simulink model "QD2_MissionCtrl_Swarm_6x_R2021a"  (R2021a)
settings: Solver=ode2  StartTime=0.0  StopTime=inf  FixedStep=0.001  RelTol=1e-3  EnableMultiTasking=on
undefined symbols (not defined in the file): datetime, Host, localhost, m, qc_get_step_size, saved_data
libraries: quarc_library x64, simulink x19, simulink_extras x1
(part 2 of 3)

== system QD2_MissionCtrl_Swarm_6x_R2021a/MISSION SERVER QDRONE SWARM/Calculate Home Pose V4 ==
  note: This subsystem waits during the first 5 seconds of starting the Mission Server before passing any post measurement.
      | This is to let the initial transient settles down (initialization, communication with the localization system, etc).
      | After the first 5 seconds, this subsystem will latch and pass along the pose measure as the QDrone Home Pose when
      | the ARM signal is received.
      | This home position will reflect whatever pose the user initially places the QDrone in.
      | This is with respect to the Research Studio Frame (RSF).
      |
      | NOTE : The height value of the home pose is the initial measured height PLUS the Home height (m) input value.
  Home height (m) : Inport
  "Pose (m, rad ) [4]" : Inport  Port=2
  Arm(0,1) : Inport  Port=3
  Clock : Clock
  Compare To Constant : simulink/Logic and Bit Operations/Compare To Constant  relop=>  const=5  OutDataTypeStr=boolean
  Constant : Constant  Value=0
  Constant1 : Constant
  Demux : Demux
  Enabled Subsystem : Subsystem  TreatAsAtomicUnit=on
  Logical Operator : Logic  AllPortsSameDT=off  OutDataTypeStr=boolean
  Mux : Mux
  One Shot : quarc_library/Discontinuities/One Shot  trigger_type=Rising edge  redun_pulse=Ignore extraneous pulse  width_source=Specify via dialog  pulse_width=1/qc_get_step_size
      settings: SourceProductName=QUARC Targets
  Selector : Selector  InputPortWidth=6  IndexOptions=Index vector (dialog)  Indices=[1:3,6]  OutputSizes=1
  Sum : Sum
  "Home Pose (m, rad) [4]" : Outport  VectorParamsAs1DForOutWhenUnconnected=off
  wires:
  Constant/1 -> One Shot/2
  Constant1/1 -> One Shot/3
  Arm(0,1)/1 -> One Shot/1
  One Shot/1 -> Logical Operator/2
  "Pose (m, rad ) [4]"/1 -> Selector/1
  Clock/1 -> Compare To Constant/1
  Compare To Constant/1 -> Logical Operator/1
  Logical Operator/1 -> Enabled Subsystem/Enable
  Enabled Subsystem/1("Home Pose (m, rad ) [4]") -> Demux/1
  Demux/1 -> Mux/1
  Demux/2 -> Mux/2
  Demux/4 -> Mux/4
  Demux/3 -> Sum/1
  Sum/1 -> Mux/3
  Home height (m)/1 -> Sum/2
  Mux/1 -> "Home Pose (m, rad) [4]"/1
  Selector/1 -> Enabled Subsystem/1("Pose (m, rad ) [4] ")

== system QD2_MissionCtrl_Swarm_6x_R2021a/MISSION SERVER QDRONE SWARM/Calculate Home Pose V5 ==
  note: This subsystem waits during the first 5 seconds of starting the Mission Server before passing any post measurement.
      | This is to let the initial transient settles down (initialization, communication with the localization system, etc).
      | After the first 5 seconds, this subsystem will latch and pass along the pose measure as the QDrone Home Pose when
      | the ARM signal is received.
      | This home position will reflect whatever pose the user initially places the QDrone in.
      | This is with respect to the Research Studio Frame (RSF).
      |
      | NOTE : The height value of the home pose is the initial measured height PLUS the Home height (m) input value.
  Home height (m) : Inport
  "Pose (m, rad ) [4]" : Inport  Port=2
  Arm(0,1) : Inport  Port=3
  Clock : Clock
  Compare To Constant : simulink/Logic and Bit Operations/Compare To Constant  relop=>  const=5  OutDataTypeStr=boolean
  Constant : Constant  Value=0
  Constant1 : Constant
  Demux : Demux
  Enabled Subsystem : Subsystem  TreatAsAtomicUnit=on
  Logical Operator : Logic  AllPortsSameDT=off  OutDataTypeStr=boolean
  Mux : Mux
  One Shot : quarc_library/Discontinuities/One Shot  trigger_type=Rising edge  redun_pulse=Ignore extraneous pulse  width_source=Specify via dialog  pulse_width=1/qc_get_step_size
      settings: SourceProductName=QUARC Targets
  Selector : Selector  InputPortWidth=6  IndexOptions=Index vector (dialog)  Indices=[1:3,6]  OutputSizes=1
  Sum : Sum
  "Home Pose (m, rad) [4]" : Outport  VectorParamsAs1DForOutWhenUnconnected=off
  wires:
  Constant/1 -> One Shot/2
  Constant1/1 -> One Shot/3
  Arm(0,1)/1 -> One Shot/1
  One Shot/1 -> Logical Operator/2
  "Pose (m, rad ) [4]"/1 -> Selector/1
  Clock/1 -> Compare To Constant/1
  Compare To Constant/1 -> Logical Operator/1
  Logical Operator/1 -> Enabled Subsystem/Enable
  Enabled Subsystem/1("Home Pose (m, rad ) [4]") -> Demux/1
  Demux/1 -> Mux/1
  Demux/2 -> Mux/2
  Demux/4 -> Mux/4
  Demux/3 -> Sum/1
  Sum/1 -> Mux/3
  Home height (m)/1 -> Sum/2
  Mux/1 -> "Home Pose (m, rad) [4]"/1
  Selector/1 -> Enabled Subsystem/1("Pose (m, rad ) [4] ")

== system QD2_MissionCtrl_Swarm_6x_R2021a/MISSION SERVER QDRONE SWARM/Calculate Home Pose V6 ==
  note: This subsystem waits during the first 5 seconds of starting the Mission Server before passing any post measurement.
      | This is to let the initial transient settles down (initialization, communication with the localization system, etc).
      | After the first 5 seconds, this subsystem will latch and pass along the pose measure as the QDrone Home Pose when
      | the ARM signal is received.
      | This home position will reflect whatever pose the user initially places the QDrone in.
      | This is with respect to the Research Studio Frame (RSF).
      |
      | NOTE : The height value of the home pose is the initial measured height PLUS the Home height (m) input value.
  Home height (m) : Inport
  "Pose (m, rad ) [4]" : Inport  Port=2
  Arm(0,1) : Inport  Port=3
  Clock : Clock
  Compare To Constant : simulink/Logic and Bit Operations/Compare To Constant  relop=>  const=5  OutDataTypeStr=boolean
  Constant : Constant  Value=0
  Constant1 : Constant
  Demux : Demux
  Enabled Subsystem : Subsystem  TreatAsAtomicUnit=on
  Logical Operator : Logic  AllPortsSameDT=off  OutDataTypeStr=boolean
  Mux : Mux
  One Shot : quarc_library/Discontinuities/One Shot  trigger_type=Rising edge  redun_pulse=Ignore extraneous pulse  width_source=Specify via dialog  pulse_width=1/qc_get_step_size
      settings: SourceProductName=QUARC Targets
  Selector : Selector  InputPortWidth=6  IndexOptions=Index vector (dialog)  Indices=[1:3,6]  OutputSizes=1
  Sum : Sum
  "Home Pose (m, rad) [4]" : Outport  VectorParamsAs1DForOutWhenUnconnected=off
  wires:
  Constant/1 -> One Shot/2
  Constant1/1 -> One Shot/3
  Arm(0,1)/1 -> One Shot/1
  One Shot/1 -> Logical Operator/2
  "Pose (m, rad ) [4]"/1 -> Selector/1
  Clock/1 -> Compare To Constant/1
  Compare To Constant/1 -> Logical Operator/1
  Logical Operator/1 -> Enabled Subsystem/Enable
  Enabled Subsystem/1("Home Pose (m, rad ) [4]") -> Demux/1
  Demux/1 -> Mux/1
  Demux/2 -> Mux/2
  Demux/4 -> Mux/4
  Demux/3 -> Sum/1
  Sum/1 -> Mux/3
  Home height (m)/1 -> Sum/2
  Mux/1 -> "Home Pose (m, rad) [4]"/1
  Selector/1 -> Enabled Subsystem/1("Pose (m, rad ) [4] ")

== system QD2_MissionCtrl_Swarm_6x_R2021a/MISSION SERVER QDRONE SWARM/Calculate Home Pose V7 ==
  note: This subsystem waits during the first 5 seconds of starting the Mission Server before passing any post measurement.
      | This is to let the initial transient settles down (initialization, communication with the localization system, etc).
      | After the first 5 seconds, this subsystem will latch and pass along the pose measure as the QDrone Home Pose when
      | the ARM signal is received.
      | This home position will reflect whatever pose the user initially places the QDrone in.
      | This is with respect to the Research Studio Frame (RSF).
      |
      | NOTE : The height value of the home pose is the initial measured height PLUS the Home height (m) input value.
  Home height (m) : Inport
  "Pose (m, rad ) [4]" : Inport  Port=2
  Arm(0,1) : Inport  Port=3
  Clock : Clock
  Compare To Constant : simulink/Logic and Bit Operations/Compare To Constant  relop=>  const=5  OutDataTypeStr=boolean
  Constant : Constant  Value=0
  Constant1 : Constant
  Demux : Demux
  Enabled Subsystem : Subsystem  TreatAsAtomicUnit=on
  Logical Operator : Logic  AllPortsSameDT=off  OutDataTypeStr=boolean
  Mux : Mux
  One Shot : quarc_library/Discontinuities/One Shot  trigger_type=Rising edge  redun_pulse=Ignore extraneous pulse  width_source=Specify via dialog  pulse_width=1/qc_get_step_size
      settings: SourceProductName=QUARC Targets
  Sum : Sum
  "Home Pose (m, rad) [4]" : Outport  VectorParamsAs1DForOutWhenUnconnected=off
  wires:
  Constant/1 -> One Shot/2
  Constant1/1 -> One Shot/3
  Arm(0,1)/1 -> One Shot/1
  One Shot/1 -> Logical Operator/2
  "Pose (m, rad ) [4]"/1 -> Enabled Subsystem/1("Pose (m, rad ) [4] ")
  Clock/1 -> Compare To Constant/1
  Compare To Constant/1 -> Logical Operator/1
  Logical Operator/1 -> Enabled Subsystem/Enable
  Enabled Subsystem/1("Home Pose (m, rad ) [4]") -> Demux/1
  Demux/1 -> Mux/1
  Demux/2 -> Mux/2
  Demux/4 -> Mux/4
  Demux/3 -> Sum/1
  Sum/1 -> Mux/3
  Home height (m)/1 -> Sum/2
  Mux/1 -> "Home Pose (m, rad) [4]"/1

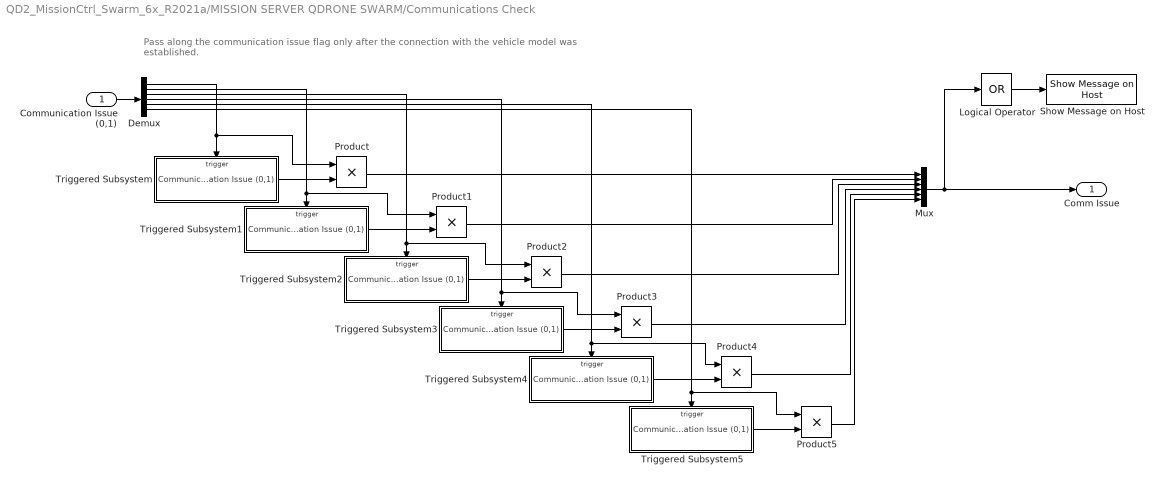
== system QD2_MissionCtrl_Swarm_6x_R2021a/MISSION SERVER QDRONE SWARM/Communications Check ==
  note: Pass along the communication issue flag only after the connection with the vehicle model was established.
  Communication Issue (0,1) : Inport
  Demux : Demux  Outputs=6
  Logical Operator : Logic  Operator=OR  Inputs=1  AllPortsSameDT=off  OutDataTypeStr=boolean
  Mux : Mux  Inputs=6
  Product{,1..5} (6 alike) : Product
  Show Message on Host : quarc_library/Sinks/Error Handling/Show Message on Host  message_type=Fixed error message  message_icon=Warning  message=Mission Server: Communication Issue with a QDrone
      settings: AttributesFormatString="\"%<message>\""  SourceProductName=QUARC Targets
  Triggered Subsystem : Subsystem  TreatAsAtomicUnit=on
  Triggered Subsystem1 : Subsystem  TreatAsAtomicUnit=on
  Triggered Subsystem2 : Subsystem  TreatAsAtomicUnit=on
  Triggered Subsystem3 : Subsystem  TreatAsAtomicUnit=on
  Triggered Subsystem4 : Subsystem  TreatAsAtomicUnit=on
  Triggered Subsystem5 : Subsystem  TreatAsAtomicUnit=on
  Comm Issue : Outport  VectorParamsAs1DForOutWhenUnconnected=off
  wires:
  Communication Issue (0,1)/1 -> Demux/1
  Demux/1 -> Product/1, Triggered Subsystem/Trigger
  Demux/2 -> Product1/1, Triggered Subsystem1/Trigger
  Demux/3 -> Product2/1, Triggered Subsystem2/Trigger
  Demux/4 -> Product3/1, Triggered Subsystem3/Trigger
  Demux/5 -> Product4/1, Triggered Subsystem4/Trigger
  Demux/6 -> Product5/1, Triggered Subsystem5/Trigger
  Triggered Subsystem/1(Communication Issue (0,1)) -> Product/2
  Triggered Subsystem5/1(Communication Issue (0,1)) -> Product5/2
  Triggered Subsystem4/1(Communication Issue (0,1)) -> Product4/2
  Triggered Subsystem3/1(Communication Issue (0,1)) -> Product3/2
  Triggered Subsystem2/1(Communication Issue (0,1)) -> Product2/2
  Triggered Subsystem1/1(Communication Issue (0,1)) -> Product1/2
  Product4/1 -> Mux/5
  Product3/1 -> Mux/4
  Product5/1 -> Mux/6
  Product2/1 -> Mux/3
  Product1/1 -> Mux/2
  Product/1 -> Mux/1
  Mux/1 -> Logical Operator/1, Comm Issue/1
  Logical Operator/1 -> Show Message on Host/1

== system QD2_MissionCtrl_Swarm_6x_R2021a/MISSION SERVER QDRONE SWARM/Extract Vehicle Data 1 ==
  Optitrack Data : Inport
  Vehicle ID : Inport  Port=2
  Data Type Conversion10 : DataTypeConversion
  Data Type Conversion11 : DataTypeConversion
  Data Type Conversion9 : DataTypeConversion
  Extract Object Data : MATLAB Function  TreatAsAtomicUnit=on
  Mux1 : Mux  Inputs=3
  Reshape : Reshape
  Reshape1 : Reshape
  Reshape2 : Reshape
  Vehicle Data : Outport  VectorParamsAs1DForOutWhenUnconnected=off
  wires:
  Reshape2/1 -> Data Type Conversion9/1
  Reshape1/1 -> Data Type Conversion10/1
  Reshape/1 -> Data Type Conversion11/1
  Data Type Conversion9/1 -> Mux1/3
  Data Type Conversion10/1 -> Mux1/2
  Data Type Conversion11/1 -> Mux1/1
  Extract Object Data/2(orientation) -> Reshape1/1
  Extract Object Data/3(tracking) -> Reshape2/1
  Extract Object Data/1(position) -> Reshape/1
  Mux1/1 -> Vehicle Data/1
  Optitrack Data/1 -> Extract Object Data/1(data)
  Vehicle ID/1 -> Extract Object Data/2(index)

== system QD2_MissionCtrl_Swarm_6x_R2021a/MISSION SERVER QDRONE SWARM/Extract Vehicle Data 2 ==
  Optitrack Data : Inport
  Vehicle ID : Inport  Port=2
  Data Type Conversion10 : DataTypeConversion
  Data Type Conversion11 : DataTypeConversion
  Data Type Conversion9 : DataTypeConversion
  Extract Object Data : MATLAB Function  TreatAsAtomicUnit=on
  Mux1 : Mux  Inputs=3
  Reshape : Reshape
  Reshape1 : Reshape
  Reshape2 : Reshape
  Vehicle Data : Outport  VectorParamsAs1DForOutWhenUnconnected=off
  wires:
  Vehicle ID/1 -> Extract Object Data/2(index)
  Optitrack Data/1 -> Extract Object Data/1(data)
  Mux1/1 -> Vehicle Data/1
  Extract Object Data/1(position) -> Reshape/1
  Extract Object Data/3(tracking) -> Reshape2/1
  Extract Object Data/2(orientation) -> Reshape1/1
  Data Type Conversion11/1 -> Mux1/1
  Data Type Conversion10/1 -> Mux1/2
  Data Type Conversion9/1 -> Mux1/3
  Reshape/1 -> Data Type Conversion11/1
  Reshape1/1 -> Data Type Conversion10/1
  Reshape2/1 -> Data Type Conversion9/1

== system QD2_MissionCtrl_Swarm_6x_R2021a/MISSION SERVER QDRONE SWARM/Extract Vehicle Data 3 ==
  Optitrack Data : Inport
  Vehicle ID : Inport  Port=2
  Data Type Conversion10 : DataTypeConversion
  Data Type Conversion11 : DataTypeConversion
  Data Type Conversion9 : DataTypeConversion
  Extract Object Data : MATLAB Function  TreatAsAtomicUnit=on
  Mux1 : Mux  Inputs=3
  Reshape : Reshape
  Reshape1 : Reshape
  Reshape2 : Reshape
  Vehicle Data : Outport  VectorParamsAs1DForOutWhenUnconnected=off
  wires:
  Vehicle ID/1 -> Extract Object Data/2(index)
  Optitrack Data/1 -> Extract Object Data/1(data)
  Mux1/1 -> Vehicle Data/1
  Extract Object Data/1(position) -> Reshape/1
  Extract Object Data/3(tracking) -> Reshape2/1
  Extract Object Data/2(orientation) -> Reshape1/1
  Data Type Conversion11/1 -> Mux1/1
  Data Type Conversion10/1 -> Mux1/2
  Data Type Conversion9/1 -> Mux1/3
  Reshape/1 -> Data Type Conversion11/1
  Reshape1/1 -> Data Type Conversion10/1
  Reshape2/1 -> Data Type Conversion9/1

== system QD2_MissionCtrl_Swarm_6x_R2021a/MISSION SERVER QDRONE SWARM/Extract Vehicle Data 4 ==
  Optitrack Data : Inport
  Vehicle ID : Inport  Port=2
  Data Type Conversion10 : DataTypeConversion
  Data Type Conversion11 : DataTypeConversion
  Data Type Conversion9 : DataTypeConversion
  Extract Object Data : MATLAB Function  TreatAsAtomicUnit=on
  Mux1 : Mux  Inputs=3
  Reshape : Reshape
  Reshape1 : Reshape
  Reshape2 : Reshape
  Vehicle Data : Outport  VectorParamsAs1DForOutWhenUnconnected=off
  wires:
  Reshape2/1 -> Data Type Conversion9/1
  Reshape1/1 -> Data Type Conversion10/1
  Reshape/1 -> Data Type Conversion11/1
  Data Type Conversion9/1 -> Mux1/3
  Data Type Conversion10/1 -> Mux1/2
  Data Type Conversion11/1 -> Mux1/1
  Extract Object Data/2(orientation) -> Reshape1/1
  Extract Object Data/3(tracking) -> Reshape2/1
  Extract Object Data/1(position) -> Reshape/1
  Mux1/1 -> Vehicle Data/1
  Optitrack Data/1 -> Extract Object Data/1(data)
  Vehicle ID/1 -> Extract Object Data/2(index)

== system QD2_MissionCtrl_Swarm_6x_R2021a/MISSION SERVER QDRONE SWARM/Extract Vehicle Data 5 ==
  Optitrack Data : Inport
  Vehicle ID : Inport  Port=2
  Data Type Conversion10 : DataTypeConversion
  Data Type Conversion11 : DataTypeConversion
  Data Type Conversion9 : DataTypeConversion
  Extract Object Data : MATLAB Function  TreatAsAtomicUnit=on
  Mux1 : Mux  Inputs=3
  Reshape : Reshape
  Reshape1 : Reshape
  Reshape2 : Reshape
  Vehicle Data : Outport  VectorParamsAs1DForOutWhenUnconnected=off
  wires:
  Vehicle ID/1 -> Extract Object Data/2(index)
  Optitrack Data/1 -> Extract Object Data/1(data)
  Mux1/1 -> Vehicle Data/1
  Extract Object Data/1(position) -> Reshape/1
  Extract Object Data/3(tracking) -> Reshape2/1
  Extract Object Data/2(orientation) -> Reshape1/1
  Data Type Conversion11/1 -> Mux1/1
  Data Type Conversion10/1 -> Mux1/2
  Data Type Conversion9/1 -> Mux1/3
  Reshape/1 -> Data Type Conversion11/1
  Reshape1/1 -> Data Type Conversion10/1
  Reshape2/1 -> Data Type Conversion9/1

== system QD2_MissionCtrl_Swarm_6x_R2021a/MISSION SERVER QDRONE SWARM/Extract Vehicle Data 6 ==
  Optitrack Data : Inport
  Vehicle ID : Inport  Port=2
  Data Type Conversion10 : DataTypeConversion
  Data Type Conversion11 : DataTypeConversion
  Data Type Conversion9 : DataTypeConversion
  Extract Object Data : MATLAB Function  TreatAsAtomicUnit=on
  Mux1 : Mux  Inputs=3
  Reshape : Reshape
  Reshape1 : Reshape
  Reshape2 : Reshape
  Vehicle Data : Outport  VectorParamsAs1DForOutWhenUnconnected=off
  wires:
  Reshape2/1 -> Data Type Conversion9/1
  Reshape1/1 -> Data Type Conversion10/1
  Reshape/1 -> Data Type Conversion11/1
  Data Type Conversion9/1 -> Mux1/3
  Data Type Conversion10/1 -> Mux1/2
  Data Type Conversion11/1 -> Mux1/1
  Extract Object Data/2(orientation) -> Reshape1/1
  Extract Object Data/3(tracking) -> Reshape2/1
  Extract Object Data/1(position) -> Reshape/1
  Mux1/1 -> Vehicle Data/1
  Optitrack Data/1 -> Extract Object Data/1(data)
  Vehicle ID/1 -> Extract Object Data/2(index)

== system QD2_MissionCtrl_Swarm_6x_R2021a/MISSION SERVER QDRONE SWARM/Extract Vehicle Data 7 ==
  Optitrack Data : Inport
  Vehicle ID : Inport  Port=2
  Data Type Conversion10 : DataTypeConversion
  Data Type Conversion11 : DataTypeConversion
  Data Type Conversion9 : DataTypeConversion
  Extract Object Data : MATLAB Function  TreatAsAtomicUnit=on
  Mux1 : Mux  Inputs=3
  Reshape : Reshape
  Reshape1 : Reshape
  Reshape2 : Reshape
  Vehicle Data : Outport  VectorParamsAs1DForOutWhenUnconnected=off
  wires:
  Reshape2/1 -> Data Type Conversion9/1
  Reshape1/1 -> Data Type Conversion10/1
  Reshape/1 -> Data Type Conversion11/1
  Data Type Conversion9/1 -> Mux1/3
  Data Type Conversion10/1 -> Mux1/2
  Data Type Conversion11/1 -> Mux1/1
  Extract Object Data/2(orientation) -> Reshape1/1
  Extract Object Data/3(tracking) -> Reshape2/1
  Extract Object Data/1(position) -> Reshape/1
  Mux1/1 -> Vehicle Data/1
  Optitrack Data/1 -> Extract Object Data/1(data)
  Vehicle ID/1 -> Extract Object Data/2(index)

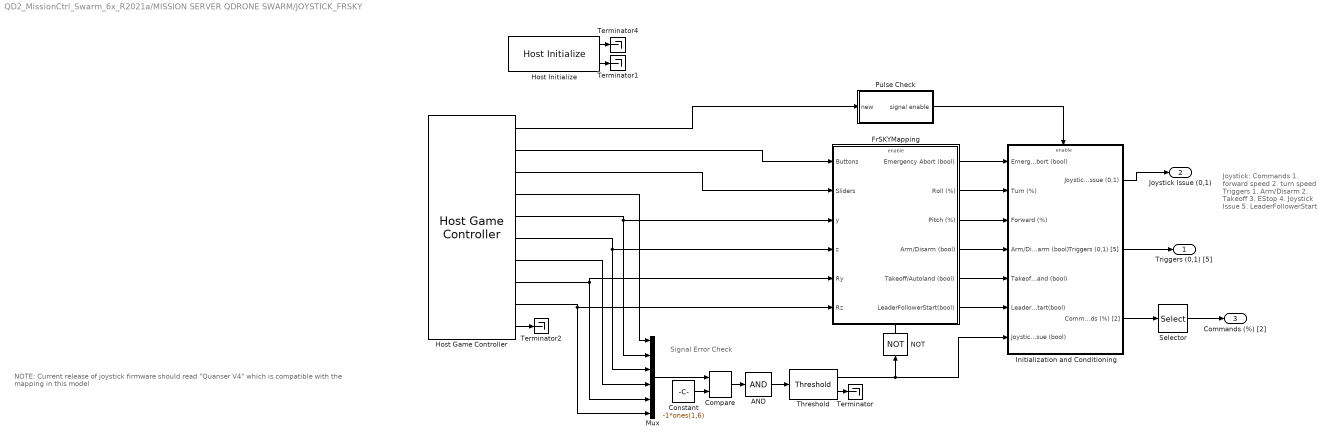
== system QD2_MissionCtrl_Swarm_6x_R2021a/MISSION SERVER QDRONE SWARM/JOYSTICK_FRSKY ==
  note: Signal Error Check
  note: NOTE: Current release of joystick firmware should read "Quanser V4" which is compatible with the mapping in this model
  note: Joystick:
      | Commands
      | 	1. forward speed
      | 	2. turn speed
      | Triggers
      | 	1. Arm/Disarm
      | 	2. Takeoff
      | 	3. EStop
      | 	4. Joystick Issue
      |
      | 	5. LeaderFollowerStart
  AND : Logic  Inputs=1  AllPortsSameDT=off  OutDataTypeStr=boolean
  Compare : quarc_library/Logic Operations/Compare  operator===  output_data_type=boolean
      settings: SourceProductName=QUARC Targets
  Constant : Constant  Value=-1*ones(1,6)
  FrSKYMapping : Subsystem
  Host Game Controller : quarc_library/Devices/Peripherals/Host/Host Game Controller  object_name=Host-1  controller=1  buffer_size=20  deadzone=[]  saturation=[]  sample_time=qc_get_step_size  auto_center=off  enabled=on  debug_mode=off
      settings: SourceProductName=QUARC Targets
  Host Initialize : quarc_library/Devices/Peripherals/Host/Host Initialize  object_name=Host-1  uri_source=Specify via dialog (do not evaluate)  uri=tcpip://localhost:18005  send_buffer_size=1000  receive_buffer_size=1000  thread_priority=0  run_client=on  use_window=off  window_position=[]  sample_time=qc_get_step_size  active=on
      settings: AttributesFormatString="\"tcpip://localhost:18005\""  SourceProductName=QUARC Targets
  Initialization and Conditioning : Subsystem  TreatAsAtomicUnit=on
  Mux : Mux  Inputs=6
  NOT : Logic  Operator=NOT  IconShape=distinctive  AllPortsSameDT=off  OutDataTypeStr=boolean
  Pulse Check : Subsystem  TreatAsAtomicUnit=on
  Selector : Selector  InputPortWidth=2  IndexOptions=Index vector (dialog)  Indices=[2 1]  OutputSizes=1
  Terminator{,1..2,4} (4 alike) : Terminator
  Threshold : quarc_library/Discontinuities/Threshold  operator=>=  param_src=Specify via dialog  threshold=0.5  duration=0.2
      settings: SourceProductName=QUARC Targets
  Triggers (0,1) [5] : Outport  VectorParamsAs1DForOutWhenUnconnected=off
  Joystick Issue (0,1) : Outport  Port=2  VectorParamsAs1DForOutWhenUnconnected=off
  Commands (%) [2] : Outport  Port=3  VectorParamsAs1DForOutWhenUnconnected=off
  wires:
  Host Game Controller/10 -> Terminator2/1
  Pulse Check/1(signal enable) -> Initialization and Conditioning/Enable
  Host Initialize/1 -> Terminator4/1
  FrSKYMapping/4("Arm/Disarm (bool) ") -> Initialization and Conditioning/4(Arm/Disarm (bool))
  Host Initialize/2 -> Terminator1/1
  FrSKYMapping/5(Takeoff/Autoland (bool)) -> Initialization and Conditioning/5(Takeoff/AutoLand (bool))
  Host Game Controller/7 -> Mux/4
  Host Game Controller/8 -> Mux/5, FrSKYMapping/5(Ry)
  Initialization and Conditioning/3(Commands (%) [2]) -> Selector/1
  Host Game Controller/5 -> Mux/2, FrSKYMapping/3(y)
  Host Game Controller/9 -> Mux/6, FrSKYMapping/6(Rz)
  Host Game Controller/1 -> Pulse Check/1(new)
  Mux/1 -> Compare/1
  Threshold/1 -> NOT/1, Initialization and Conditioning/7(Joystick Issue (bool))
  AND/1 -> Threshold/1
  Host Game Controller/3 -> FrSKYMapping/2(Sliders)
  Threshold/2 -> Terminator/1
  NOT/1 -> FrSKYMapping/Enable
  Constant/1 -> Compare/2
  Host Game Controller/6 -> Mux/3, FrSKYMapping/4(z)
  FrSKYMapping/2(Roll (%)) -> Initialization and Conditioning/2(Turn (%))
  FrSKYMapping/3(Pitch (%)) -> Initialization and Conditioning/3(Forward (%))
  Compare/1 -> AND/1
  FrSKYMapping/1(Emergency Abort (bool)) -> Initialization and Conditioning/1(Emergency Abort (bool))
  Initialization and Conditioning/1(Joystick Issue (0,1)) -> Joystick Issue (0,1)/1
  Initialization and Conditioning/2(Triggers (0,1) [5]) -> Triggers (0,1) [5]/1
  Host Game Controller/4 -> Mux/1
  Host Game Controller/2 -> FrSKYMapping/1(Buttons)
  FrSKYMapping/6(LeaderFollowerStart(bool)) -> Initialization and Conditioning/6(LeaderFollowerStart(bool))
  Selector/1 -> Commands (%) [2]/1

== system QD2_MissionCtrl_Swarm_6x_R2021a/MISSION SERVER QDRONE SWARM/JOYSTICK_SPEKTRUM ==
  note: Throttle
      | Roll
      | Pitch
      | Yaw
  Host Game Controller : quarc_library/Devices/Peripherals/Host/Host Game Controller  object_name=Host-2  controller=1  buffer_size=20  deadzone=[]  saturation=[]  sample_time=qc_get_step_size  auto_center=off  enabled=on  debug_mode=off
      settings: SourceProductName=QUARC Targets
  Host Initialize : quarc_library/Devices/Peripherals/Host/Host Initialize  object_name=Host-2  uri_source=Use external mode communications  uri=tcpip://localhost:18001  send_buffer_size=1000  receive_buffer_size=1000  thread_priority=0  run_client=on  use_window=off  window_position=[]  sample_time=qc_get_step_size  active=on
      settings: SourceProductName=QUARC Targets
  Initialization and Conditioning : Subsystem  TreatAsAtomicUnit=on
  Pulse Check : Subsystem  TreatAsAtomicUnit=on
  Spectrum DXe Mapping : Subsystem
  Terminator{1..4} (4 alike) : Terminator
  Triggers (0,1) [4] : Outport  VectorParamsAs1DForOutWhenUnconnected=off
  Joystick Issue (0,1) : Outport  Port=2  VectorParamsAs1DForOutWhenUnconnected=off
  Commands (%) [4] : Outport  Port=3  VectorParamsAs1DForOutWhenUnconnected=off
  wires:
  Pulse Check/1(signal enable) -> Initialization and Conditioning/Enable
  Host Game Controller/1 -> Pulse Check/1(new), Spectrum DXe Mapping/1(new)
  Initialization and Conditioning/3(Commands (%) [4]) -> Commands (%) [4]/1
  Spectrum DXe Mapping/8(Takeoff/Autoland (bool)) -> Initialization and Conditioning/8(Takeoff/AutoLand (bool))
  Initialization and Conditioning/2(Triggers (0,1) [4]) -> Triggers (0,1) [4]/1
  Spectrum DXe Mapping/2(Emergency Abort (bool)) -> Initialization and Conditioning/2(Emergency Abort (bool))
  Host Game Controller/2 -> Spectrum DXe Mapping/2(buttons)
  Spectrum DXe Mapping/6(Pitch (%)) -> Initialization and Conditioning/6(Pitch (%))
  Spectrum DXe Mapping/4(Throttle (%)) -> Initialization and Conditioning/4(Throttle (%))
  Spectrum DXe Mapping/5(Roll (%)) -> Initialization and Conditioning/5(Roll (%))
  Spectrum DXe Mapping/7("Arm/Disarm (bool) ") -> Initialization and Conditioning/7(Arm/Disarm (bool))
  Spectrum DXe Mapping/3(Yaw (%)) -> Initialization and Conditioning/3(Yaw (%))
  Host Initialize/2 -> Terminator1/1
  Host Initialize/1 -> Terminator4/1
  Host Game Controller/6 -> Spectrum DXe Mapping/6(z)
  Host Game Controller/3 -> Spectrum DXe Mapping/3(Sliders)
  Host Game Controller/5 -> Spectrum DXe Mapping/5(y)
  Host Game Controller/4 -> Spectrum DXe Mapping/4(x)
  Host Game Controller/8 -> Spectrum DXe Mapping/8(Ry)
  Host Game Controller/9 -> Terminator2/1
  Host Game Controller/10 -> Terminator3/1
  Host Game Controller/7 -> Spectrum DXe Mapping/7(Rx)
  Spectrum DXe Mapping/1(Joystick Issue (bool)) -> Initialization and Conditioning/1(Joystick Issue (bool))
  Initialization and Conditioning/1(Joystick Issue (0,1)) -> Joystick Issue (0,1)/1

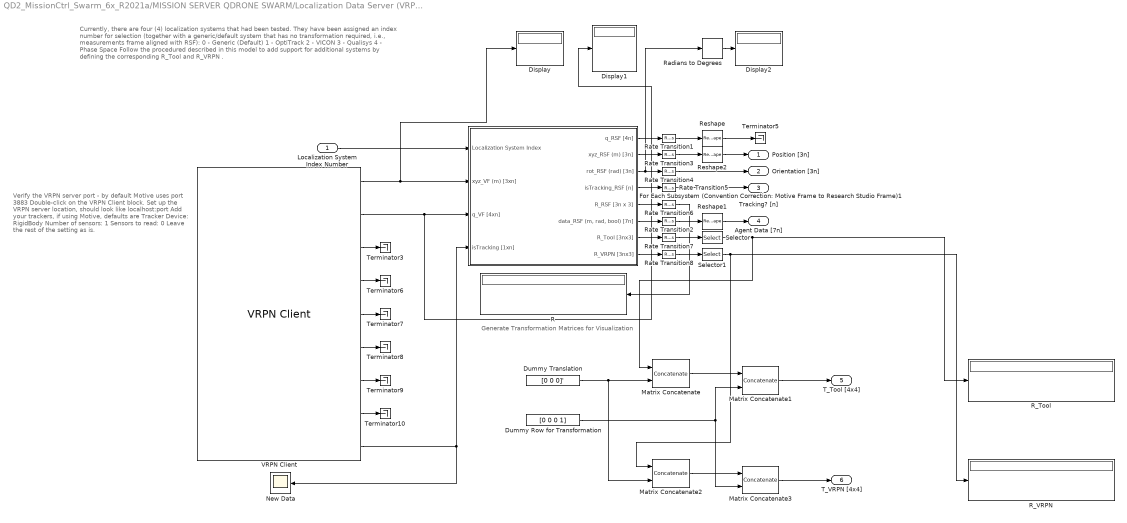
== system QD2_MissionCtrl_Swarm_6x_R2021a/MISSION SERVER QDRONE SWARM/Localization Data Server (VRPN)  ==
  note: Generate Transformation Matrices for Visualization
  note: Verify the VRPN server port - by default Motive uses port 3883
      | Double-click on the VRPN Client block.
      |
      | Set up the VRPN server location, should look like
      | localhost:port
      |
      | Add your trackers,
      | if using Motive, defaults are
      | Tracker Device: RigidBody
      | Number of sensors: 1
      | Sensors to read: 0
      |
      | Leave the rest of the setting as is.
  note: Currently, there are four (4) localization systems that had been tested. They have been assigned an index number for selection (together with a generic/default system that has no transformation required, i.e., measurements frame aligned with RSF):
      |
      | 0 - Generic (Default)
      | 1 - OptiTrack
      | 2 - VICON
      | 3 - Qualisys
      | 4 - Phase Space
      |
      | Follow the procedured described in this model to add support for additional systems by defining the corresponding R_Tool and R_VRPN .
  Localization System Index Number : Inport
  Display : Display
  Display1 : Display
  Display2 : Display
  Dummy Row for Transformation : Constant  Value=[0 0 0 1]  VectorParams1D=off
  Dummy Translation : Constant  Value=[0 0 0]'  VectorParams1D=off
  For Each Subsystem (Convention Correction: Motive Frame to Research Studio Frame)1 : Subsystem  TreatAsAtomicUnit=on
  Matrix Concatenate : Concatenate  Mode=Multidimensional array  ConcatenateDimension=2
  Matrix Concatenate1 : Concatenate  Mode=Multidimensional array
  Matrix Concatenate2 : Concatenate  Mode=Multidimensional array  ConcatenateDimension=2
  Matrix Concatenate3 : Concatenate  Mode=Multidimensional array
  New Data : Scope
  R : Display
  R_Tool : Display
  R_VRPN : Display
  Radians to Degrees : simulink_extras/Transformations/Radians to Degrees
  Rate Transition{1..8} (8 alike) : RateTransition
  Reshape : Reshape
  Reshape1 : Reshape
  Reshape2 : Reshape
  Selector : Selector  NumberOfDimensions=2  InputPortWidth=3  IndexOptions=Index vector (dialog),Index vector (dialog)  Indices=[1:3],[1:3]  OutputSizes=1,1
  Selector1 : Selector  NumberOfDimensions=2  InputPortWidth=3  IndexOptions=Index vector (dialog),Index vector (dialog)  Indices=[1:3],[1:3]  OutputSizes=1,1
  Terminator{3,5..10} (7 alike) : Terminator
  VRPN Client : quarc_library/Devices/Third-Party/VRPN/VRPN Client  server_address=localhost:3883  trackerstable={ 'RigidBody1', '1', '0'; 'RigidBody2', '1', '0'; 'RigidBody3', '1', '0'; 'RigidBody4', '1', '0'; 'RigidBody5', '1', '0'; 'RigidBody6', '1', '0' }  trackers_list_mask='RigidBody1|RigidBody2|RigidBody3|RigidBody4|RigidBody5|RigidBody6'  trackers_num_sensors="[1  1  1  1  1  1]"  trackers_sensors_to_read_arg="[1  1  1  1  1  1  0  0  0  0  0  0]"  trackers_jpl=off  sample_time=qc_get_step_size*16  active=on
      settings: SourceProductName=QUARC Targets
  Position [3n] : Outport  VectorParamsAs1DForOutWhenUnconnected=off
  Orientation [3n] : Outport  Port=2  VectorParamsAs1DForOutWhenUnconnected=off
  Tracking? [n] : Outport  Port=3  VectorParamsAs1DForOutWhenUnconnected=off
  Agent Data [7n] : Outport  Port=4  VectorParamsAs1DForOutWhenUnconnected=off
  T_Tool [4x4] : Outport  Port=5  VectorParamsAs1DForOutWhenUnconnected=off
  T_VRPN [4x4] : Outport  Port=6  VectorParamsAs1DForOutWhenUnconnected=off
  wires:
  VRPN Client/1 -> Display/1, For Each Subsystem (Convention Correction: Motive Frame to Research Studio Frame)1/2(xyz_VF (m) [3xn])
  VRPN Client/2 -> Display1/1, For Each Subsystem (Convention Correction: Motive Frame to Research Studio Frame)1/3(q_VF [4xn])
  For Each Subsystem (Convention Correction: Motive Frame to Research Studio Frame)1/4(isTracking_RSF [n]) -> Rate Transition5/1
  For Each Subsystem (Convention Correction: Motive Frame to Research Studio Frame)1/3(rot_RSF (rad) [3n]) -> Radians to Degrees/1, Rate Transition4/1
  For Each Subsystem (Convention Correction: Motive Frame to Research Studio Frame)1/2(xyz_RSF (m) [3n]) -> Rate Transition3/1
  VRPN Client/3 -> Terminator3/1
  Reshape/1 -> Terminator5/1
  VRPN Client/4 -> Terminator6/1
  VRPN Client/5 -> Terminator7/1
  VRPN Client/6 -> Terminator8/1
  VRPN Client/7 -> Terminator9/1
  VRPN Client/8 -> Terminator10/1
  VRPN Client/9 -> For Each Subsystem (Convention Correction: Motive Frame to Research Studio Frame)1/4(isTracking [1xn]), New Data/1
  For Each Subsystem (Convention Correction: Motive Frame to Research Studio Frame)1/6("data_RSF (m, rad, bool) [7n]") -> Rate Transition2/1
  For Each Subsystem (Convention Correction: Motive Frame to Research Studio Frame)1/1(q_RSF [4n]) -> Rate Transition1/1
  Rate Transition2/1 -> Reshape1/1
  Rate Transition1/1 -> Reshape/1
  Reshape1/1 -> Agent Data [7n]/1
  Reshape2/1 -> Position [3n]/1
  Rate Transition3/1 -> Reshape2/1
  Rate Transition4/1 -> Orientation [3n]/1
  Rate Transition5/1 -> Tracking? [n]/1
  For Each Subsystem (Convention Correction: Motive Frame to Research Studio Frame)1/5(R_RSF [3n x 3]) -> Rate Transition6/1
  Rate Transition6/1 -> R/1
  Localization System Index Number/1 -> For Each Subsystem (Convention Correction: Motive Frame to Research Studio Frame)1/1(Localization System Index)
  For Each Subsystem (Convention Correction: Motive Frame to Research Studio Frame)1/7(R_Tool [3nx3]) -> Rate Transition7/1
  Rate Transition7/1 -> Selector/1
  Rate Transition8/1 -> Selector1/1
  For Each Subsystem (Convention Correction: Motive Frame to Research Studio Frame)1/8(R_VRPN [3nx3]) -> Rate Transition8/1
  Selector/1 -> Matrix Concatenate/1, R_Tool/1
  Dummy Translation/1 -> Matrix Concatenate2/2, Matrix Concatenate/2
  Matrix Concatenate/1 -> Matrix Concatenate1/1
  Matrix Concatenate1/1 -> T_Tool [4x4]/1
  Dummy Row for Transformation/1 -> Matrix Concatenate3/2, Matrix Concatenate1/2
  Matrix Concatenate2/1 -> Matrix Concatenate3/1
  Selector1/1 -> Matrix Concatenate2/1, R_VRPN/1
  Matrix Concatenate3/1 -> T_VRPN [4x4]/1
  Radians to Degrees/1 -> Display2/1

== system QD2_MissionCtrl_Swarm_6x_R2021a/MISSION SERVER QDRONE SWARM/Measurement Conditioning 1 ==
  note: Position and Position Rate Estimates Conditioning
  Data : Inport
  Data Type Conversion : DataTypeConversion
  Data Type Conversion1 : DataTypeConversion
  Data Type Conversion2 : DataTypeConversion
  Demux : Demux  Outputs=[3 3 1]
  Mux : Mux  Inputs=2
  Mux2 : Mux  Inputs=2
  Saturation : Saturate  UpperLimit=[2 2 3]  LowerLimit=[-2 -2 0]
  Selector : Selector  InputPortWidth=3  IndexOptions=Index vector (dialog)  Indices=[3]  OutputSizes=1
  Selector1 : Selector  InputPortWidth=3  IndexOptions=Index vector (dialog)  Indices=[1,2]  OutputSizes=1
  Subtract Rigid Body Reference Offset (Initial Height) to get height above the ground : Bias  Bias=[0 0 -0.07]
  Unwrap optitrack measurement : quarc_library/Discontinuities/Inverse Modulus  modulus=2*pi  output_derivative=off  output_revolutions=off  max_x=Inf  min_x=-Inf
  "Measured Pose (m, rad) [6]" : Outport  VectorParamsAs1DForOutWhenUnconnected=off
  isTracking : Outport  Port=2  VectorParamsAs1DForOutWhenUnconnected=off
  wires:
  Demux/2 -> Data Type Conversion1/1
  Demux/1 -> Data Type Conversion/1
  Demux/3 -> Data Type Conversion2/1
  Mux2/1 -> "Measured Pose (m, rad) [6]"/1
  Data/1 -> Demux/1
  Data Type Conversion2/1 -> isTracking/1
  Subtract Rigid Body Reference Offset (Initial Height) to get height above the ground/1 -> Saturation/1
  Saturation/1 -> Mux2/1
  Data Type Conversion1/1 -> Selector1/1, Selector/1
  Selector/1 -> Unwrap optitrack measurement/1
  Data Type Conversion/1 -> Subtract Rigid Body Reference Offset (Initial Height) to get height above the ground/1
  Unwrap optitrack measurement/1 -> Mux/2  "1"
  Mux/1 -> Mux2/2
  Selector1/1 -> Mux/1  "2"

== system QD2_MissionCtrl_Swarm_6x_R2021a/MISSION SERVER QDRONE SWARM/Measurement Conditioning 2 ==
  note: Position and Position Rate Estimates Conditioning
  Data : Inport
  Data Type Conversion : DataTypeConversion
  Data Type Conversion1 : DataTypeConversion
  Data Type Conversion2 : DataTypeConversion
  Demux : Demux  Outputs=[3 3 1]
  Mux : Mux  Inputs=2
  Mux2 : Mux  Inputs=2
  Saturation : Saturate  UpperLimit=[2 2 3]  LowerLimit=[-2 -2 0]
  Selector : Selector  InputPortWidth=3  IndexOptions=Index vector (dialog)  Indices=[3]  OutputSizes=1
  Selector1 : Selector  InputPortWidth=3  IndexOptions=Index vector (dialog)  Indices=[1,2]  OutputSizes=1
  Subtract Rigid Body Reference Offset (Initial Height) to get height above the ground : Bias  Bias=[0 0 -0.07]
  Unwrap optitrack measurement : quarc_library/Discontinuities/Inverse Modulus  modulus=2*pi  output_derivative=off  output_revolutions=off  max_x=Inf  min_x=-Inf
  "Measured Pose (m, rad) [6]" : Outport  VectorParamsAs1DForOutWhenUnconnected=off
  isTracking : Outport  Port=2  VectorParamsAs1DForOutWhenUnconnected=off
  wires:
  Demux/2 -> Data Type Conversion1/1
  Demux/1 -> Data Type Conversion/1
  Demux/3 -> Data Type Conversion2/1
  Mux2/1 -> "Measured Pose (m, rad) [6]"/1
  Data/1 -> Demux/1
  Data Type Conversion2/1 -> isTracking/1
  Subtract Rigid Body Reference Offset (Initial Height) to get height above the ground/1 -> Saturation/1
  Saturation/1 -> Mux2/1
  Data Type Conversion1/1 -> Selector1/1, Selector/1
  Selector/1 -> Unwrap optitrack measurement/1
  Data Type Conversion/1 -> Subtract Rigid Body Reference Offset (Initial Height) to get height above the ground/1
  Unwrap optitrack measurement/1 -> Mux/2  "1"
  Mux/1 -> Mux2/2
  Selector1/1 -> Mux/1  "2"

== system QD2_MissionCtrl_Swarm_6x_R2021a/MISSION SERVER QDRONE SWARM/Measurement Conditioning 3 ==
  note: Position and Position Rate Estimates Conditioning
  Data : Inport
  Data Type Conversion : DataTypeConversion
  Data Type Conversion1 : DataTypeConversion
  Data Type Conversion2 : DataTypeConversion
  Demux : Demux  Outputs=[3 3 1]
  Mux : Mux  Inputs=2
  Mux2 : Mux  Inputs=2
  Saturation : Saturate  UpperLimit=[2 2 3]  LowerLimit=[-2 -2 0]
  Selector : Selector  InputPortWidth=3  IndexOptions=Index vector (dialog)  Indices=[3]  OutputSizes=1
  Selector1 : Selector  InputPortWidth=3  IndexOptions=Index vector (dialog)  Indices=[1,2]  OutputSizes=1
  Subtract Rigid Body Reference Offset (Initial Height) to get height above the ground : Bias  Bias=[0 0 -0.07]
  Unwrap optitrack measurement : quarc_library/Discontinuities/Inverse Modulus  modulus=2*pi  output_derivative=off  output_revolutions=off  max_x=Inf  min_x=-Inf
  "Measured Pose (m, rad) [6]" : Outport  VectorParamsAs1DForOutWhenUnconnected=off
  isTracking : Outport  Port=2  VectorParamsAs1DForOutWhenUnconnected=off
  wires:
  Demux/2 -> Data Type Conversion1/1
  Demux/1 -> Data Type Conversion/1
  Demux/3 -> Data Type Conversion2/1
  Mux2/1 -> "Measured Pose (m, rad) [6]"/1
  Data/1 -> Demux/1
  Data Type Conversion2/1 -> isTracking/1
  Subtract Rigid Body Reference Offset (Initial Height) to get height above the ground/1 -> Saturation/1
  Saturation/1 -> Mux2/1
  Data Type Conversion1/1 -> Selector1/1, Selector/1
  Selector/1 -> Unwrap optitrack measurement/1
  Data Type Conversion/1 -> Subtract Rigid Body Reference Offset (Initial Height) to get height above the ground/1
  Unwrap optitrack measurement/1 -> Mux/2  "1"
  Mux/1 -> Mux2/2
  Selector1/1 -> Mux/1  "2"

== system QD2_MissionCtrl_Swarm_6x_R2021a/MISSION SERVER QDRONE SWARM/Measurement Conditioning 4 ==
  note: Position and Position Rate Estimates Conditioning
  Data : Inport
  Data Type Conversion : DataTypeConversion
  Data Type Conversion1 : DataTypeConversion
  Data Type Conversion2 : DataTypeConversion
  Demux : Demux  Outputs=[3 3 1]
  Mux : Mux  Inputs=2
  Mux2 : Mux  Inputs=2
  Saturation : Saturate  UpperLimit=[2 2 3]  LowerLimit=[-2 -2 0]
  Selector : Selector  InputPortWidth=3  IndexOptions=Index vector (dialog)  Indices=[3]  OutputSizes=1
  Selector1 : Selector  InputPortWidth=3  IndexOptions=Index vector (dialog)  Indices=[1,2]  OutputSizes=1
  Subtract Rigid Body Reference Offset (Initial Height) to get height above the ground : Bias  Bias=[0 0 -0.07]
  Unwrap optitrack measurement : quarc_library/Discontinuities/Inverse Modulus  modulus=2*pi  output_derivative=off  output_revolutions=off  max_x=Inf  min_x=-Inf
  "Measured Pose (m, rad) [6]" : Outport  VectorParamsAs1DForOutWhenUnconnected=off
  isTracking : Outport  Port=2  VectorParamsAs1DForOutWhenUnconnected=off
  wires:
  Demux/2 -> Data Type Conversion1/1
  Demux/1 -> Data Type Conversion/1
  Demux/3 -> Data Type Conversion2/1
  Mux2/1 -> "Measured Pose (m, rad) [6]"/1
  Data/1 -> Demux/1
  Data Type Conversion2/1 -> isTracking/1
  Subtract Rigid Body Reference Offset (Initial Height) to get height above the ground/1 -> Saturation/1
  Saturation/1 -> Mux2/1
  Data Type Conversion1/1 -> Selector1/1, Selector/1
  Selector/1 -> Unwrap optitrack measurement/1
  Data Type Conversion/1 -> Subtract Rigid Body Reference Offset (Initial Height) to get height above the ground/1
  Unwrap optitrack measurement/1 -> Mux/2  "1"
  Mux/1 -> Mux2/2
  Selector1/1 -> Mux/1  "2"

== system QD2_MissionCtrl_Swarm_6x_R2021a/MISSION SERVER QDRONE SWARM/Measurement Conditioning 5 ==
  note: Position and Position Rate Estimates Conditioning
  Data : Inport
  Data Type Conversion : DataTypeConversion
  Data Type Conversion1 : DataTypeConversion
  Data Type Conversion2 : DataTypeConversion
  Demux : Demux  Outputs=[3 3 1]
  Mux : Mux  Inputs=2
  Mux2 : Mux  Inputs=2
  Saturation : Saturate  UpperLimit=[2 2 3]  LowerLimit=[-2 -2 0]
  Selector : Selector  InputPortWidth=3  IndexOptions=Index vector (dialog)  Indices=[3]  OutputSizes=1
  Selector1 : Selector  InputPortWidth=3  IndexOptions=Index vector (dialog)  Indices=[1,2]  OutputSizes=1
  Subtract Rigid Body Reference Offset (Initial Height) to get height above the ground : Bias  Bias=[0 0 -0.07]
  Unwrap optitrack measurement : quarc_library/Discontinuities/Inverse Modulus  modulus=2*pi  output_derivative=off  output_revolutions=off  max_x=Inf  min_x=-Inf
  "Measured Pose (m, rad) [6]" : Outport  VectorParamsAs1DForOutWhenUnconnected=off
  isTracking : Outport  Port=2  VectorParamsAs1DForOutWhenUnconnected=off
  wires:
  Demux/2 -> Data Type Conversion1/1
  Demux/1 -> Data Type Conversion/1
  Demux/3 -> Data Type Conversion2/1
  Mux2/1 -> "Measured Pose (m, rad) [6]"/1
  Data/1 -> Demux/1
  Data Type Conversion2/1 -> isTracking/1
  Subtract Rigid Body Reference Offset (Initial Height) to get height above the ground/1 -> Saturation/1
  Saturation/1 -> Mux2/1
  Data Type Conversion1/1 -> Selector1/1, Selector/1
  Selector/1 -> Unwrap optitrack measurement/1
  Data Type Conversion/1 -> Subtract Rigid Body Reference Offset (Initial Height) to get height above the ground/1
  Unwrap optitrack measurement/1 -> Mux/2  "1"
  Mux/1 -> Mux2/2
  Selector1/1 -> Mux/1  "2"

== system QD2_MissionCtrl_Swarm_6x_R2021a/MISSION SERVER QDRONE SWARM/Measurement Conditioning 6 ==
  note: Position and Position Rate Estimates Conditioning
  Data : Inport
  Data Type Conversion : DataTypeConversion
  Data Type Conversion1 : DataTypeConversion
  Data Type Conversion2 : DataTypeConversion
  Demux : Demux  Outputs=[3 3 1]
  Mux : Mux  Inputs=2
  Mux2 : Mux  Inputs=2
  Saturation : Saturate  UpperLimit=[2 2 3]  LowerLimit=[-2 -2 0]
  Selector : Selector  InputPortWidth=3  IndexOptions=Index vector (dialog)  Indices=[3]  OutputSizes=1
  Selector1 : Selector  InputPortWidth=3  IndexOptions=Index vector (dialog)  Indices=[1,2]  OutputSizes=1
  Subtract Rigid Body Reference Offset (Initial Height) to get height above the ground : Bias  Bias=[0 0 -0.07]
  Unwrap optitrack measurement : quarc_library/Discontinuities/Inverse Modulus  modulus=2*pi  output_derivative=off  output_revolutions=off  max_x=Inf  min_x=-Inf
  "Measured Pose (m, rad) [6]" : Outport  VectorParamsAs1DForOutWhenUnconnected=off
  isTracking : Outport  Port=2  VectorParamsAs1DForOutWhenUnconnected=off
  wires:
  Demux/2 -> Data Type Conversion1/1
  Demux/1 -> Data Type Conversion/1
  Demux/3 -> Data Type Conversion2/1
  Mux2/1 -> "Measured Pose (m, rad) [6]"/1
  Data/1 -> Demux/1
  Data Type Conversion2/1 -> isTracking/1
  Subtract Rigid Body Reference Offset (Initial Height) to get height above the ground/1 -> Saturation/1
  Saturation/1 -> Mux2/1
  Data Type Conversion1/1 -> Selector1/1, Selector/1
  Selector/1 -> Unwrap optitrack measurement/1
  Data Type Conversion/1 -> Subtract Rigid Body Reference Offset (Initial Height) to get height above the ground/1
  Unwrap optitrack measurement/1 -> Mux/2  "1"
  Mux/1 -> Mux2/2
  Selector1/1 -> Mux/1  "2"

== system QD2_MissionCtrl_Swarm_6x_R2021a/MISSION SERVER QDRONE SWARM/Measurement Conditioning 7 ==
  note: Position and Position Rate Estimates Conditioning
  Data : Inport
  Data Type Conversion : DataTypeConversion
  Data Type Conversion1 : DataTypeConversion
  Data Type Conversion2 : DataTypeConversion
  Demux : Demux  Outputs=[3 3 1]
  Mux2 : Mux  Inputs=[3 1]
  Saturation : Saturate  UpperLimit=[2 2 3]  LowerLimit=[-2 -2 0]
  Selector : Selector  InputPortWidth=3  IndexOptions=Index vector (dialog)  Indices=[3]  OutputSizes=1
  Subtract Rigid Body Reference Offset (Initial Height) to get height above the ground : Bias  Bias=[0 0 -0.07]
  Unwrap optitrack measurement : quarc_library/Discontinuities/Inverse Modulus  modulus=2*pi  output_derivative=off  output_revolutions=off  max_x=Inf  min_x=-Inf
  "Measured Pose (m, rad) [4]" : Outport  VectorParamsAs1DForOutWhenUnconnected=off
  isTracking : Outport  Port=2  VectorParamsAs1DForOutWhenUnconnected=off
  wires:
  Demux/2 -> Data Type Conversion1/1
  Demux/1 -> Data Type Conversion/1
  Demux/3 -> Data Type Conversion2/1
  Mux2/1 -> "Measured Pose (m, rad) [4]"/1
  Data/1 -> Demux/1
  Data Type Conversion2/1 -> isTracking/1
  Subtract Rigid Body Reference Offset (Initial Height) to get height above the ground/1 -> Saturation/1
  Saturation/1 -> Mux2/1
  Data Type Conversion1/1 -> Selector/1
  Selector/1 -> Unwrap optitrack measurement/1
  Data Type Conversion/1 -> Subtract Rigid Body Reference Offset (Initial Height) to get height above the ground/1
  Unwrap optitrack measurement/1 -> Mux2/2

== system QD2_MissionCtrl_Swarm_6x_R2021a/MISSION SERVER QDRONE SWARM/calculate loop back time ==
  Timestamp sent (s) : Inport
  Timestamps received (s) [6] : Inport  Port=2
  Demux : Demux  Outputs=6
  Mux : Mux  Inputs=6
  Subtract{,1..5} (6 alike) : Sum  Inputs=+-
  Loop Back Tmes (s) [6] : Outport  VectorParamsAs1DForOutWhenUnconnected=off
  wires:
  Timestamp sent (s)/1 -> Subtract1/1, Subtract2/1, Subtract3/1, Subtract4/1, Subtract5/1, Subtract/1
  Timestamps received (s) [6]/1 -> Demux/1
  Demux/1 -> Subtract/2
  Demux/2 -> Subtract1/2
  Demux/3 -> Subtract2/2
  Demux/4 -> Subtract3/2
  Demux/5 -> Subtract4/2
  Demux/6 -> Subtract5/2
  Subtract/1 -> Mux/1
  Subtract1/1 -> Mux/2
  Subtract2/1 -> Mux/3
  Subtract3/1 -> Mux/4
  Subtract4/1 -> Mux/5
  Subtract5/1 -> Mux/6
  Mux/1 -> Loop Back Tmes (s) [6]/1

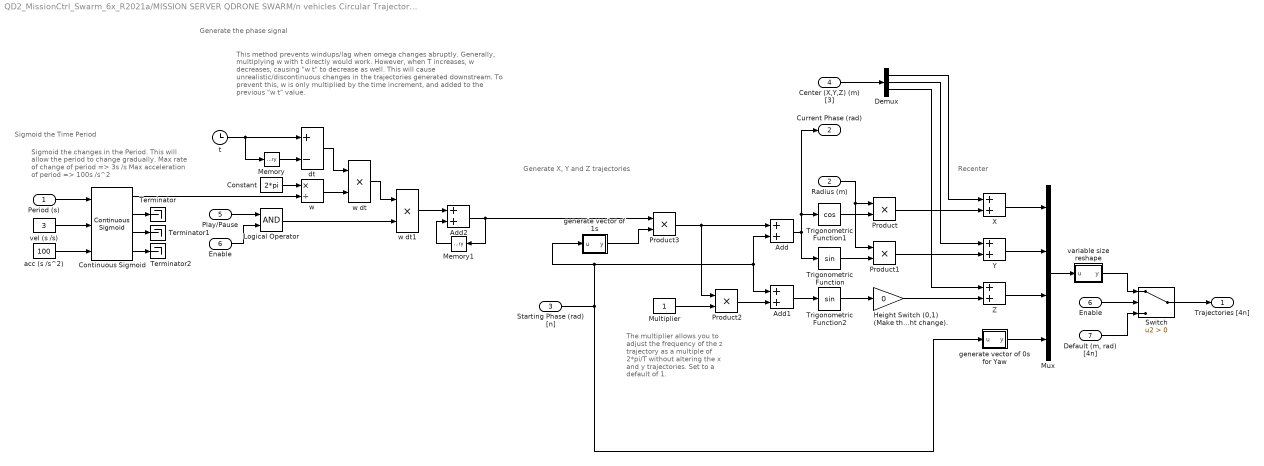
== system QD2_MissionCtrl_Swarm_6x_R2021a/MISSION SERVER QDRONE SWARM/n vehicles Circular Trajectories ==
  note: Recenter
  note: Generate X, Y and Z trajectories
  note: Generate the phase signal
  note: Sigmoid the changes in the Period. This will
      | allow the period to change gradually.
      | Max rate of change of period => 3s /s
      | Max acceleration of period => 100s /s^2
  note: Sigmoid the Time Period
  note: The multiplier allows you to adjust the frequency of the z trajectory as a multiple of 2*pi/T without altering the x and y trajectories. Set to a default of 1.
  note: This method prevents windups/lag when omega changes abruptly. Generally, multiplying w with t directly would work. However, when T increases, w decreases, causing "w t" to decrease as well. This will cause unrealistic/discontinuous changes in the trajectories generated downstream.
      |
      | To prevent this, w is only multiplied by the time increment, and added to the previous "w t" value.
  Period (s) : Inport
  Radius (m) : Inport  Port=2
  Starting Phase (rad) [n] : Inport  Port=3
  Center (X,Y,Z) (m) [3] : Inport  Port=4
  Play/Pause : Inport  Port=5
  Enable : Inport  Port=6
  "Default (m, rad) [4n]" : Inport  Port=7
  " Enable " : InportShadow  Port=6
  Add : Sum
  Add1 : Sum
  Add2 : Sum
  Constant : Constant  Value=2*pi
  Continuous Sigmoid : quarc_library/Sources/Sigmoids/Continuous Sigmoid  params_source=External (input ports)  max_velocity=2  max_acceleration=10  initial_position=10  initial_velocity=0  hold_off=0.5  input_sample_time=-1  output_sample_time=qc_get_step_size
      settings: SourceProductName=QUARC Targets
  Demux : Demux  Outputs=3
  Height Switch (0,1) (Make this 0 to disable height change). : Gain  Gain=0
  Logical Operator : Logic  AllPortsSameDT=off  OutDataTypeStr=boolean
  Memory : Memory
  Memory1 : Memory
  Multiplier : Constant
  Mux : Mux
  Product{,1..3} (4 alike) : Product
  Switch : Switch  Criteria=u2 > Threshold
  Terminator : Terminator
  Terminator1 : Terminator
  Terminator2 : Terminator
  Trigonometric Function : Trigonometry
  Trigonometric Function1 : Trigonometry  Operator=cos
  Trigonometric Function2 : Trigonometry
  X : Sum
  Y : Sum
  Z : Sum
  acc (s /s^2) : Constant  Value=100
  dt : Sum  Inputs=+-
  generate vector of 0s for Yaw : MATLAB Function  TreatAsAtomicUnit=on
  generate vector of 1s : MATLAB Function  TreatAsAtomicUnit=on
  t : Clock
  variable size reshape : MATLAB Function  TreatAsAtomicUnit=on
  vel (s /s) : Constant  Value=3
  w : Product  Inputs=*/
  w dt : Product
  w dt1 : Product
  Trajectories [4n] : Outport  VectorParamsAs1DForOutWhenUnconnected=off
  Current Phase (rad) : Outport  Port=2  VectorParamsAs1DForOutWhenUnconnected=off
  wires:
  Trigonometric Function/1 -> Product1/2
  Trigonometric Function1/1 -> Product/2
  Height Switch (0,1) (Make this 0 to disable height change)./1 -> Z/2
  Product1/1 -> Y/2
  Product/1 -> X/2
  Radius (m)/1 -> Product/1, Product1/1
  generate vector of 0s for Yaw/1(y) -> Mux/4
  Continuous Sigmoid/4 -> Terminator2/1
  Period (s)/1 -> Continuous Sigmoid/1
  Continuous Sigmoid/2 -> Terminator/1
  Continuous Sigmoid/3 -> Terminator1/1
  acc (s /s^2)/1 -> Continuous Sigmoid/3
  vel (s /s)/1 -> Continuous Sigmoid/2
  Add1/1 -> Trigonometric Function2/1
  Multiplier/1 -> Product2/2
  Starting Phase (rad) [n]/1 -> generate vector of 1s/1(u), Add/2, Add1/1, generate vector of 0s for Yaw/1(u)
  Add2/1 -> Product3/1, Memory1/1
  Add/1 -> Current Phase (rad)/1, Trigonometric Function1/1, Trigonometric Function/1
  Center (X,Y,Z) (m) [3]/1 -> Demux/1
  Demux/2 -> Y/1
  Demux/1 -> X/1
  Trigonometric Function2/1 -> Height Switch (0,1) (Make this 0 to disable height change)./1
  Demux/3 -> Z/1
  X/1 -> Mux/1
  Y/1 -> Mux/2
  Z/1 -> Mux/3
  Memory/1 -> dt/2
  w dt/1 -> w dt1/1
  w dt1/1 -> Add2/1
  Constant/1 -> w/1
  Memory1/1 -> Add2/2
  w/1 -> w dt/2
  Continuous Sigmoid/1 -> w/2
  t/1 -> Memory/1, dt/1
  dt/1 -> w dt/1
  Mux/1 -> variable size reshape/1(u)
  Switch/1 -> Trajectories [4n]/1
  "Default (m, rad) [4n]"/1 -> Switch/3
  Enable/1 -> Switch/2
  Play/Pause/1 -> Logical Operator/1
  " Enable "/1 -> Logical Operator/2
  Logical Operator/1 -> w dt1/2
  Product3/1 -> Add/1, Product2/1
  variable size reshape/1(y) -> Switch/1
  generate vector of 1s/1(y) -> Product3/2
  Product2/1 -> Add1/2

== system QD2_MissionCtrl_Swarm_6x_R2021a/MISSION SERVER QDRONE SWARM/Calculate Home Pose V1/Enabled Subsystem ==
  "Pose (m, rad ) [4] " : Inport
  Enable : EnablePort
  "Home Pose (m, rad ) [4]" : Outport  VectorParamsAs1DForOutWhenUnconnected=off
  wires:
  "Pose (m, rad ) [4] "/1 -> "Home Pose (m, rad ) [4]"/1

== system QD2_MissionCtrl_Swarm_6x_R2021a/MISSION SERVER QDRONE SWARM/Calculate Home Pose V2/Enabled Subsystem ==
  "Pose (m, rad ) [4] " : Inport
  Enable : EnablePort
  "Home Pose (m, rad ) [4]" : Outport  VectorParamsAs1DForOutWhenUnconnected=off
  wires:
  "Pose (m, rad ) [4] "/1 -> "Home Pose (m, rad ) [4]"/1

== system QD2_MissionCtrl_Swarm_6x_R2021a/MISSION SERVER QDRONE SWARM/Calculate Home Pose V3/Enabled Subsystem ==
  "Pose (m, rad ) [4] " : Inport
  Enable : EnablePort
  "Home Pose (m, rad ) [4]" : Outport  VectorParamsAs1DForOutWhenUnconnected=off
  wires:
  "Pose (m, rad ) [4] "/1 -> "Home Pose (m, rad ) [4]"/1

== system QD2_MissionCtrl_Swarm_6x_R2021a/MISSION SERVER QDRONE SWARM/Calculate Home Pose V4/Enabled Subsystem ==
  "Pose (m, rad ) [4] " : Inport
  Enable : EnablePort
  "Home Pose (m, rad ) [4]" : Outport  VectorParamsAs1DForOutWhenUnconnected=off
  wires:
  "Pose (m, rad ) [4] "/1 -> "Home Pose (m, rad ) [4]"/1

== system QD2_MissionCtrl_Swarm_6x_R2021a/MISSION SERVER QDRONE SWARM/Calculate Home Pose V5/Enabled Subsystem ==
  "Pose (m, rad ) [4] " : Inport
  Enable : EnablePort
  "Home Pose (m, rad ) [4]" : Outport  VectorParamsAs1DForOutWhenUnconnected=off
  wires:
  "Pose (m, rad ) [4] "/1 -> "Home Pose (m, rad ) [4]"/1
